simulink model "Portantiolo250184_Assign2_EX_2"  (R2023b)
settings: Solver=ode15s  StartTime=0.0  StopTime=tf  RelTol=1e-10  AbsTol=1e-10
values from neighbouring files (symbols this model uses):
  ba = var(1)    [Portantiolo250184_Assign2_EX2.m]
  k_acc = 1    [Portantiolo250184_Assign2_EX2.m]
  k_v = 1e3    (= 1000)    [Portantiolo250184_Assign2_EX2.m]
  m_a = 0.32    [Portantiolo250184_Assign2_EX2.m]
  m_sc = 300    [Portantiolo250184_Assign2_EX2.m]
  m_v = 0.1    [Portantiolo250184_Assign2_EX2.m]
  Rf = var(4)    [Portantiolo250184_Assign2_EX2.m]
  Rin = var(3)    [Portantiolo250184_Assign2_EX2.m]
libraries: fl_lib x15, nesl_utility x7, ee_lib x1
settings Model: Creator=matteoportantiolo  LastModifiedBy=matteoportantiolo

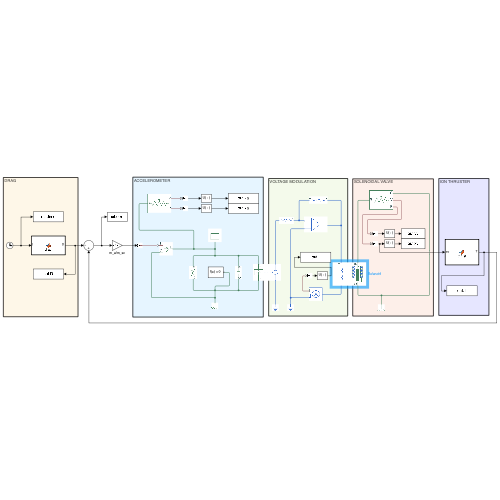
[thumbnail: Simulink's stored preview of the top-level diagram]
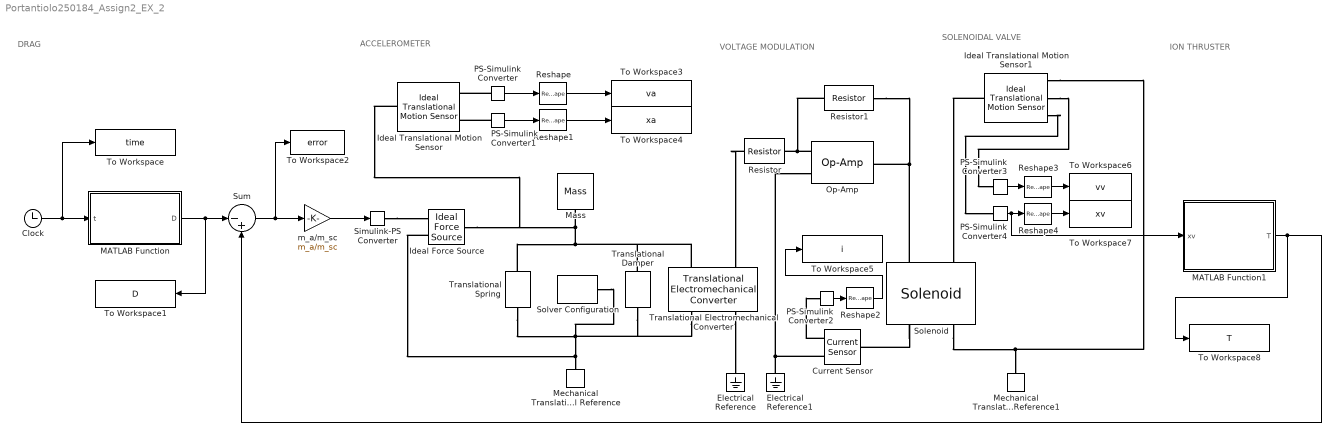
== system Portantiolo250184_Assign2_EX_2 ==
  note: ION THRUSTER
  note: SOLENOIDAL VALVE
  note: DRAG
  note: VOLTAGE MODULATION
  note: ACCELEROMETER
  Clock : Clock
  Current Sensor : fl_lib/Electrical/Electrical Sensors/Current Sensor
  Electrical Reference : fl_lib/Electrical/Electrical Elements/Electrical Reference
  Electrical Reference1 : fl_lib/Electrical/Electrical Elements/Electrical Reference
  Ideal Force Source : fl_lib/Mechanical/Mechanical Sources/Ideal Force Source
  Ideal Translational Motion Sensor : fl_lib/Mechanical/Mechanical Sensors/Ideal Translational Motion Sensor  reference=foundation.enum.MeasurementReference.absolute  acceleration_port=false  velocity_port=true  position_port=true  offset=0 m
      settings: InternalSimscapePortConfiguration="{\"Bottom\":[],\"Left\":[{\"id\":\"R\",\"label\":\"R\",\"type\":\"foundation.mechanical.translational.translational\"}],\"Right\":[{\"id\":\"V\",\"label\":\"V\",\"type\":\"output\"},{\"id\":\"P\",\"label\":\"P\",\"type\":\"output\"}],\"Top\":[]}"
  Ideal Translational Motion Sensor1 : fl_lib/Mechanical/Mechanical Sensors/Ideal Translational Motion Sensor  reference=foundation.enum.MeasurementReference.difference  acceleration_port=false  velocity_port=true  position_port=true  offset=0 m
  MATLAB Function : MATLAB Function  TreatAsAtomicUnit=on
  MATLAB Function1 : MATLAB Function  TreatAsAtomicUnit=on
  Mass : fl_lib/Mechanical/Translational Elements/Mass  mass=m_a kg  num_ports=foundation.enum.numPorts2.one  v_specify=off  v_priority=High  v=0 m/s  v_nominal_specify=off  v_nominal_unit=m/s  v_nominal_value=1  f_specify=off  f_priority=None  f=0 N  f_nominal_specify=off  f_nominal_unit=N  f_nominal_value=1
  Mechanical Translational Reference : fl_lib/Mechanical/Translational Elements/Mechanical Translational Reference
  Mechanical Translational Reference1 : fl_lib/Mechanical/Translational Elements/Mechanical Translational Reference
  Op-Amp : fl_lib/Electrical/Electrical Elements/Op-Amp  outI_specify=off  outI_priority=None  outI=0 A  outI_nominal_specify=off  outI_nominal_unit=A  outI_nominal_value=1
  PS-Simulink Converter{,1..4} (5 alike) : nesl_utility/PS-Simulink Converter  PhysicalDomain=network_engine_domain  SubClassName=ps_output  LeftPortType=input  RightPortType=output  PseudoPeriodic=off  Frequencies=[]  VectorFormat=inherit  Unit=inherit  AffineConversion=off
  Reshape{,1..4} (5 alike) : Reshape
  Resistor : fl_lib/Electrical/Electrical Elements/Resistor  R=Rin Ohm  i_specify=off  i_priority=None  i=0 A  i_nominal_specify=off  i_nominal_unit=A  i_nominal_value=1  v_specify=off  v_priority=None  v=0 V  v_nominal_specify=off  v_nominal_unit=V  v_nominal_value=1
  Resistor1 : fl_lib/Electrical/Electrical Elements/Resistor  R=Rf Ohm  i_specify=off  i_priority=None  i=0 A  i_nominal_specify=off  i_nominal_unit=A  i_nominal_value=1  v_specify=off  v_priority=None  v=0 V  v_nominal_specify=off  v_nominal_unit=V  v_nominal_value=1
  Simulink-PS Converter : nesl_utility/Simulink-PS Converter  PhysicalDomain=network_engine_domain  SubClassName=ps_input  LeftPortType=input  RightPortType=output  PseudoPeriodic=off  Frequencies=[]  NoiseDistribution=none  NoiseParameters=[]  Unit=1  AffineConversion=off  FilteringAndDerivatives=provide  SimscapeFilterOrder=1  InputFilterTimeConstant=0.001  UdotUserProvided=0
  Solenoid : ee_lib/Electromechanical/Mechatronic Actuators/Solenoid  motionDirection=ee.enum.actuators.solenoidDirection.away  F12=[9000, 12] N  X12=[0, 0.1] mm  Vdc=0.6 mV  Imax=0.1 A  K=k_v N/m  Xzero=0 mm  lam=b_v N*s/m  Mass=m_v kg  Xmax=0.1 mm  K_endstop=0.12e6 N/m  D_endstop=1e4 N*s/m  i_specify=off  i_priority=High  i=0 A  i_nominal_specify=off  i_nominal_unit=A  i_nominal_value=1  x_specify=on  x_priority=High  x=l mm  x_nominal_specify=off  x_nominal_unit=mm  x_nominal_value=1  vel_specify=off  vel_priority=None  vel=0 mm/s  vel_nominal_specify=off  vel_nominal_unit=mm/s  vel_nominal_value=1  F_specify=off  F_priority=None  F=0 N  F_nominal_specify=off  F_nominal_unit=N  F_nominal_value=1  v_L_specify=off  v_L_priority=None  v_L=0 V  v_L_nominal_specify=off  v_L_nominal_unit=V  v_L_nominal_value=1  magnetic_force_specify=off  magnetic_force_priority=None  magnetic_force=0 N  magnetic_force_nominal_specify=off  magnetic_force_nominal_unit=N  magnetic_force_nominal_value=1  alpha=3.93e-3 1/K  Tmeas=25 degC  thermal_mass=100 J/K  temperature_specify=off  temperature_priority=High  temperature=25 degC  temperature_nominal_specify=off  temperature_nominal_unit=degC  temperature_nominal_value=1  Q_specify=off  Q_priority=None  Q=0 W  Q_nominal_specify=off  Q_nominal_unit=W  Q_nominal_value=1
      settings: InternalSimscapePortConfiguration="{\"Bottom\":[],\"Left\":[{\"id\":\"p\",\"label\":\"+\",\"type\":\"foundation.electrical.electrical\"},{\"id\":\"R\",\"label\":\"R\",\"type\":\"foundation.mechanical.translational.translational\"}],\"Right\":[{\"id\":\"n\",\"label\":\"-\",\"type\":\"foundation.electrical.electrical\"},{\"id\":\"C\",\"label\":\"C\",\"type\":\"foundation.mechanical.translational.translational\"}],\"Top\":[]}"
  Solver Configuration : nesl_utility/Solver Configuration  PhysicalDomain=network_engine_domain  SubClassName=solver  LeftPortType=input  RightPortType=generic  Tones=[]  Harmonics=[]  SimulateNoise=off  Profile=off  UseLocalSampling=off  EnableSwitchedLinearOptims=on  FrequencyDomain=off  UseCCode=off  RelTol=0.001  AbsTol=0.001  MinStep=1e-09  ToWorkspace=off  RevertToSquareIcSolve=off  NumHomotopyIterations=100  PhasorMode=off  PhasorModeNumHarmonics=1  ConsistencySolver=NEWTON_XTOL_AFTER_FTOL  IndexReductionMethod=DerivativeReplacement  DoDC=off  ResidualTolerance=1e-09  ConsistencyTolSource=GLOBAL  ConsistencyAbsTol=0.001  ConsistencyRelTol=0.001  ConsistencyTolFactor=0.001  UseLocalSolver=off  LocalSolverChoice=NE_BACKWARD_EULER_ADVANCER  ResolveIndetEquations=on  FunctionEvalNumThread=1  LocalSolverSampleTime=0.001  DoFixedCost=off  MaxNonlinIter=3  MaxModeIter=2  ComputeImpulses=off  ImpulseIterations=2  LinearAlgebra=auto  LinearAlgebraNumThread=0  EquationFormulation=NE_TIME_EF  DelaysMemoryBudget=1024  AutomaticFiltering=on  FilteringTimeConstant=0.001  PartitionStorageMethod=AS_NEEDED  PartitionMemoryBudget=1024  PartitionMethod=ROBUST  MultibodyUseLocalSolver=off  MultibodyLocalSolverChoice=ODE1  MultibodyLocalSolverSampleTime=0.001
  Sum : Sum  Inputs=|-+
  To Workspace : ToWorkspace  VariableName=time  SampleTime=-1
  To Workspace1 : ToWorkspace  VariableName=D  SampleTime=-1
  To Workspace2 : ToWorkspace  VariableName=error  SampleTime=-1
  To Workspace3 : ToWorkspace  VariableName=va  SampleTime=-1
  To Workspace4 : ToWorkspace  VariableName=xa  SampleTime=-1
  To Workspace5 : ToWorkspace  VariableName=i  SampleTime=-1
  To Workspace6 : ToWorkspace  VariableName=vv  SampleTime=-1
  To Workspace7 : ToWorkspace  VariableName=xv  SampleTime=-1
  To Workspace8 : ToWorkspace  VariableName=T  SampleTime=-1
  Translational Electromechanical Converter : fl_lib/Electrical/Electrical Elements/Translational Electromechanical Converter  K=k_acc V*s/m  i_specify=off  i_priority=None  i=0 A  i_nominal_specify=off  i_nominal_unit=A  i_nominal_value=1  v_specify=off  v_priority=None  v=0 V  v_nominal_specify=off  v_nominal_unit=V  v_nominal_value=1  f_specify=off  f_priority=None  f=0 N  f_nominal_specify=off  f_nominal_unit=N  f_nominal_value=1  u_specify=off  u_priority=None  u=0 m/s  u_nominal_specify=off  u_nominal_unit=m/s  u_nominal_value=1
      settings: InternalSimscapePortConfiguration="{\"Bottom\":[],\"Left\":[{\"id\":\"p\",\"label\":\"+\",\"type\":\"foundation.electrical.electrical\"},{\"id\":\"R\",\"label\":\"R\",\"type\":\"foundation.mechanical.translational.translational\"}],\"Right\":[{\"id\":\"n\",\"label\":\"-\",\"type\":\"foundation.electrical.electrical\"},{\"id\":\"C\",\"label\":\"C\",\"type\":\"foundation.mechanical.translational.translational\"}],\"Top\":[]}"
  Translational Damper : fl_lib/Mechanical/Translational Elements/Translational Damper  D=ba N*s/m  v_specify=off  v_priority=None  v=0 m/s  v_nominal_specify=off  v_nominal_unit=m/s  v_nominal_value=1  f_specify=off  f_priority=None  f=0 N  f_nominal_specify=off  f_nominal_unit=N  f_nominal_value=1
  Translational Spring : fl_lib/Mechanical/Translational Elements/Translational Spring  spr_rate=ka N/m  v_specify=off  v_priority=None  v=0 m/s  v_nominal_specify=off  v_nominal_unit=m/s  v_nominal_value=1  f_specify=off  f_priority=None  f=0 N  f_nominal_specify=off  f_nominal_unit=N  f_nominal_value=1  x_specify=off  x_priority=High  x=0 m  x_nominal_specify=off  x_nominal_unit=m  x_nominal_value=1
  m_a/m_sc : Gain  Gain=m_a/m_sc
  wires:
  Clock/1 -> To Workspace/1, MATLAB Function/1(t)
  MATLAB Function/1(D) -> To Workspace1/1, Sum/1
  Sum/1 -> To Workspace2/1, m_a/m_sc/1
  m_a/m_sc/1 -> Simulink-PS Converter/1
  PS-Simulink Converter/1 -> Reshape/1
  PS-Simulink Converter1/1 -> Reshape1/1
  Reshape/1 -> To Workspace3/1
  Reshape1/1 -> To Workspace4/1
  PS-Simulink Converter2/1 -> Reshape2/1
  Reshape2/1 -> To Workspace5/1
  Reshape4/1 -> To Workspace7/1
  PS-Simulink Converter4/1 -> MATLAB Function1/1(xv), Reshape4/1
  Reshape3/1 -> To Workspace6/1
  PS-Simulink Converter3/1 -> Reshape3/1
  MATLAB Function1/1(T) -> Sum/2, To Workspace8/1
  connections:
  Simulink-PS Converter/RConn1 -- Ideal Force Source/RConn1
  Translational Spring/LConn1 -- Translational Electromechanical Converter/LConn2 -- Translational Damper/LConn1 -- Ideal Translational Motion Sensor/LConn1 -- Ideal Force Source/LConn1 -- Mass/LConn1
  Translational Spring/RConn1 -- Solver Configuration/RConn1 -- Translational Electromechanical Converter/RConn2 -- Translational Damper/RConn1 -- Ideal Force Source/RConn2 -- Mechanical Translational Reference/LConn1
  PS-Simulink Converter/LConn1 -- Ideal Translational Motion Sensor/RConn1
  PS-Simulink Converter1/LConn1 -- Ideal Translational Motion Sensor/RConn2
  Resistor/LConn1 -- Translational Electromechanical Converter/LConn1
  Op-Amp/LConn2 -- Resistor1/LConn1 -- Resistor/RConn1
  Solenoid/LConn1 -- Resistor1/RConn1 -- Op-Amp/RConn1
  Solenoid/RConn1 -- Current Sensor/LConn1
  Translational Electromechanical Converter/RConn1 -- Electrical Reference/LConn1
  Electrical Reference1/LConn1 -- Current Sensor/RConn2 -- Op-Amp/LConn1
  Current Sensor/RConn1 -- PS-Simulink Converter2/LConn1
  Ideal Translational Motion Sensor1/LConn1 -- Solenoid/LConn2
  Solenoid/RConn2 -- Ideal Translational Motion Sensor1/RConn1 -- Mechanical Translational Reference1/LConn1
  Ideal Translational Motion Sensor1/RConn2 -- PS-Simulink Converter3/LConn1
  Ideal Translational Motion Sensor1/RConn3 -- PS-Simulink Converter4/LConn1

== matlab function Portantiolo250184_Assign2_EX_2/MATLAB Function ==
  data: t input; D output
function D = drag(t)

% Drag
omega_s = 1.658226e-6;
omega0 = 1.160758e-3;

% Compute Drag
D = (2.2 - cos(omega_s.*t) + 1.2.*sin(omega0.*t).*cos(omega0.*t)) * 1e-3;

== matlab function Portantiolo250184_Assign2_EX_2/MATLAB Function1 ==
  data: xv input; T output
function T = thrust(xv)

% Solenoid Valve
A0 = 4.7e-12;
l = 1e-5;

% Thruster
k = 1.66;
p_t = 2e5;
T_t = 240;
R = 63.32754;
q = 1.6e-19;
dV = 2000;
m_i = 2.188e-25;

% Compute Thrust
Av = A0 + l*(l-xv);
rho = p_t / (R*T_t);
m_dot = Av * sqrt( k*rho*p_t * (2/(k+1))^((k+1)/(k-1)) );
T = m_dot * sqrt(2*q*dV/m_i);
